simulink model "first"  (R2021a)
settings: Solver=FixedStepAuto  StartTime=0.0  StopTime=150  FixedStep=0.1  RelTol=1e-3
(part 2 of 2)

== matlab function first/MATLAB Function5 ==
  data: u1 input; phi output; u2 input; u3 input; theta output; psai output
function [phi, theta, psai] = fcn(u1, u2, u3)

    phi = rem(u1,2*pi);
    theta = rem(u2,2*pi);
    psai = rem(u3,2*pi);
end

== matlab function first/Position2 ==
  data: Ux input; U1 output; Uy input; Uz input; psaid input; m input; phid output; thetad output
function [U1,phid,thetad] = fcn(Ux,Uy,Uz,psaid,m)
    U1 = m*sqrt(Ux^2+Uy^2+(Uz+9.81)^2);
    phid = asin((Ux*sin(psaid)-Uy*cos(psaid))*m/U1);
%     thetad = asin((Ux*m-U1*sin(psaid)*sin(phid))/(U1*cos(psaid)*cos(phid)));
thetad=atan((Ux*cos(psaid)+Uy*sin(psaid))/(Uz+9.81));
end

== matlab function first/MATLAB Function6 ==
  data: U1 input; w1 output; U2 input; U3 input; U4 input; w2 output; w3 output; w4 output
function [w1,w2,w3,w4] = fcn(U1,U2,U3,U4)
    CT = 1.116e-5; dCT = 0.225*CT;
    matrixA = [CT,CT,CT,CT;0,CT,0,-CT;-CT,0,CT,0;-dCT,dCT,-dCT,dCT];
    w_2 = inv(matrixA)*[U1,U2,U3,U4]';
    w1 = sqrt(abs(w_2(1))); w2 = sqrt(abs(w_2(2)));
    w3 = sqrt(abs(w_2(3))); w4 = sqrt(abs(w_2(4)));
end

== matlab function first/MATLAB Function ==
  data: U1 input; w1 output; U2 input; U3 input; U4 input; w2 output; w3 output; w4 output
function [w1,w2,w3,w4] = fcn(U1,U2,U3,U4)
    CT = 1.116e-5; dCT = 0.225*CT;
    matrixA = [CT,CT,CT,CT;0,CT,0,-CT;-CT,0,CT,0;-dCT,dCT,-dCT,dCT];
    w_2 = inv(matrixA)*[U1,U2,U3,U4]';
    w1 = sqrt(abs(w_2(1))); w2 = sqrt(abs(w_2(2)));
    w3 = sqrt(abs(w_2(3))); w4 = sqrt(abs(w_2(4)));
end

== matlab function first/MATLAB Function7 ==
  data: u1 input; phi output; u2 input; u3 input; theta output; psai output
function [phi,theta,psai] = fcn(u1,u2,u3)
    phi = rem(u1,2*pi);
    theta = rem(u2,2*pi);
    psai = rem(u3,2*pi);
end

== matlab function first/Position3 ==
  data: Ux input; U1 output; Uy input; Uz input; psaid input; m input; phid output; thetad output
function [U1,phid,thetad] = fcn(Ux,Uy,Uz,psaid,m)
    U1 = m*sqrt(Ux^2+Uy^2+(Uz+9.81)^2);
    phid = asin((Ux*sin(psaid)-Uy*cos(psaid))*m/U1);
    %thetad = asin((Ux*m-U1*sin(psaid)*sin(phid))/(U1*cos(psaid)*cos(phid)));
    thetad=atan((Ux*cos(psaid)+Uy*sin(psaid))/(Uz+9.81));
end

== matlab function first/Position ==
  data: Ux input; U1 output; Uy input; Uz input; psaid input; m input; phid output; thetad output
function [U1,phid,thetad] = fcn(Ux,Uy,Uz,psaid,m)
    U1 = m*sqrt(Ux^2+Uy^2+(Uz+9.81)^2);
    phid = asin((Ux*sin(psaid)-Uy*cos(psaid))*m/U1);
    %thetad = asin((Ux*m-U1*sin(psaid)*sin(phid))/(U1*cos(psaid)*cos(phid)));
    thetad=atan((Ux*cos(psaid)+Uy*sin(psaid))/(Uz+9.81));
end

== matlab function first/MATLAB Function1 ==
  data: u1 input; phi output; u2 input; u3 input; theta output; psai output
function [phi,theta,psai] = fcn(u1,u2,u3)
    phi = rem(u1,2*pi);
    theta = rem(u2,2*pi);
    psai = rem(u3,2*pi);
end

== matlab function first/MATLAB Function2 ==
  data: U1 input; w1 output; U2 input; U3 input; U4 input; w2 output; w3 output; w4 output
function [w1,w2,w3,w4] = fcn(U1,U2,U3,U4)
    CT = 1.116e-5; dCT = 0.225*CT;
    matrixA = [CT,CT,CT,CT;0,CT,0,-CT;-CT,0,CT,0;-dCT,dCT,-dCT,dCT];
    w_2 = inv(matrixA)*[U1,U2,U3,U4]';
    w1 = sqrt(abs(w_2(1))); w2 = sqrt(abs(w_2(2)));
    w3 = sqrt(abs(w_2(3))); w4 = sqrt(abs(w_2(4)));
end

== matlab function first/MATLAB Function3 ==
  data: u1 input; phi output; u2 input; u3 input; theta output; psai output
function [phi, theta, psai] = fcn(u1, u2, u3)

    phi = rem(u1,2*pi);
    theta = rem(u2,2*pi);
    psai = rem(u3,2*pi);
end

== matlab function first/Position1 ==
  data: Ux input; U1 output; Uy input; Uz input; psaid input; m input; phid output; thetad output
function [U1,phid,thetad] = fcn(Ux,Uy,Uz,psaid,m)
    U1 = m*sqrt(Ux^2+Uy^2+(Uz+9.81)^2);
    phid = asin((Ux*sin(psaid)-Uy*cos(psaid))*m/U1);
%     thetad = asin((Ux*m-U1*sin(psaid)*sin(phid))/(U1*cos(psaid)*cos(phid)));
thetad=atan((Ux*cos(psaid)+Uy*sin(psaid))/(Uz+9.81));
end

== matlab function first/MATLAB Function4 ==
  data: U1 input; w1 output; U2 input; U3 input; U4 input; w2 output; w3 output; w4 output
function [w1,w2,w3,w4] = fcn(U1,U2,U3,U4)
    CT = 1.116e-5; dCT = 0.225*CT;
    matrixA = [CT,CT,CT,CT;0,CT,0,-CT;-CT,0,CT,0;-dCT,dCT,-dCT,dCT];
    w_2 = inv(matrixA)*[U1,U2,U3,U4]';
    w1 = sqrt(abs(w_2(1))); w2 = sqrt(abs(w_2(2)));
    w3 = sqrt(abs(w_2(3))); w4 = sqrt(abs(w_2(4)));
end
